simulink model "sampleModel1768_sub"  (R2023a)
settings: Solver=VariableStepAuto  StartTime=0.0  StopTime=10.0  RelTol=1e-3
libraries: hdlsllib x6, simulink x2
settings Model: Creator=user1  LastModifiedBy=user1
settings OptimizationCC: BlockReduction=off  ConditionallyExecuteInputs=off

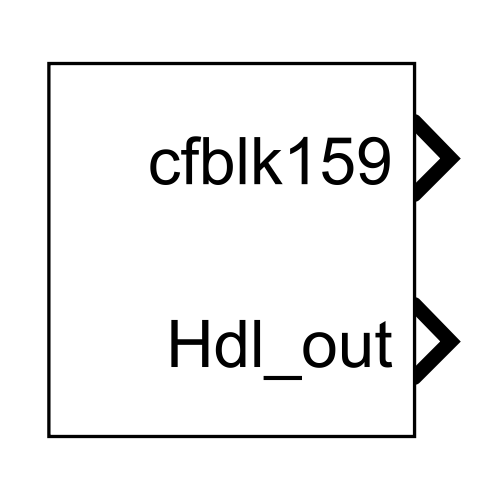
[thumbnail: Simulink's stored preview of the top-level diagram]
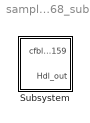
== system sampleModel1768_sub ==
  Subsystem : Subsystem

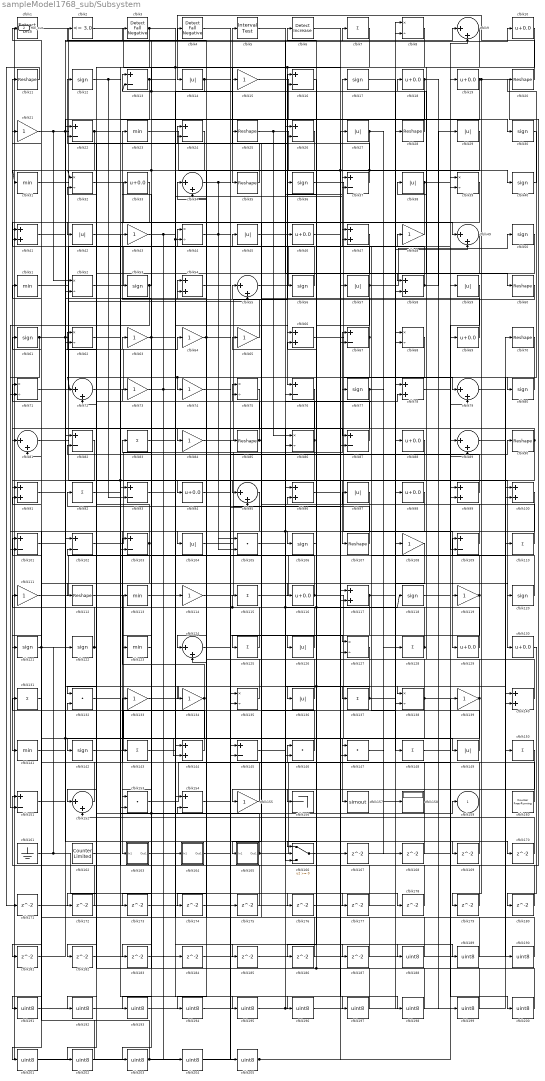
== system sampleModel1768_sub/Subsystem ==
  cfblk1 : simulink/Logic and Bit Operations/Extract Bits  bitsToExtract=Upper half  numBits=8  bitIdxRange=[0 7]  outScalingMode=Preserve fixed-point scaling
      settings: LibrarySourceBlock=|
      | hdlsllib/Logic and Bit
      | Operations/Extract Bits
  cfblk{10,18..19,33,46,69,88,94,98,116,129..130} (12 alike) : Bias  Bias=0.0  SaturateOnIntegerOverflow=off
  cfblk{41,47,54,58,66,78,91,96,99..100,117,140,144} (13 alike) : Sum  OutDataTypeStr=uint8
  cfblk{13,16,22,24,26,37,67,76,82,87,93,101..103,109,145,151,154} (18 alike) : Sum  Inputs=+-  OutDataTypeStr=uint8
  cfblk{14,27,29,38,42,45,57,59,97,104,126,136,149} (13 alike) : Abs  OutDataTypeStr=uint8  SaturateOnIntegerOverflow=off
  cfblk{105,132,146..147,153} (5 alike) : DotProduct  OutDataTypeStr=uint8
  cfblk{12,17,30,36,40,50,53,56,61,77,80,106,118,120..122,142} (17 alike) : Signum
  cfblk{11,20,25,28,35,60,70,85,90,107,112} (11 alike) : Reshape
  cfblk{15,21,43,48,63..65,73..74,84,108,111,114,119,133..134,139,155} (18 alike) : Gain  OutDataTypeStr=uint8
  cfblk{7,83,92,110,115,125,128,131,137,143,148,150} (12 alike) : Sum  Inputs=+  OutDataTypeStr=uint8
  cfblk{23,31,51,113,123,141} (6 alike) : MinMax  OutDataTypeStr=uint8
  cfblk{9,34,49,55,72,79,81,89,95,124,152} (11 alike) : Sum  Inputs=|++  OutDataTypeStr=uint8
  cfblk{8,32,39,44,52,62,68,71,75,86,127,135,138} (13 alike) : Product  Inputs=*/  OutDataTypeStr=uint8  RndMeth=Zero  SaturateOnIntegerOverflow=on
  cfblk156 : Terminator
  cfblk157 : ToWorkspace  VariableName=simout  SaveFormat=Timeseries  SampleTime=-1
  cfblk158 : Display
  cfblk160 : hdlsllib/Sources/Counter Free-Running  NumBits=16  tsamp=-1
  cfblk161 : Ground
  cfblk162 : hdlsllib/Sources/Counter Limited  uplimit=7  tsamp=-1
  cfblk163 : Subsystem
      settings: LibrarySourceBlock=|
      | hdlsllib/Ports &
      | Subsystems/Subsystem
  cfblk164 : Subsystem
      settings: LibrarySourceBlock=|
      | hdlsllib/Ports &
      | Subsystems/Subsystem
  cfblk165 : Subsystem
      settings: LibrarySourceBlock=|
      | hdlsllib/Ports &
      | Subsystems/Subsystem
  cfblk166 : Switch  OutDataTypeStr=uint8  SaturateOnIntegerOverflow=off  InputSameDT=off
  cfblk{167..187} (21 alike) : Delay  SampleTime=1
  cfblk{188..205} (18 alike) : DataTypeConversion  OutDataTypeStr=uint8  SaturateOnIntegerOverflow=off  RndMeth=Floor
  cfblk2 : hdlsllib/Logic and Bit Operations/Compare To Constant  relop=<=  const=3.0  OutDataTypeStr=uint8
  cfblk3 : hdlsllib/Logic and Bit Operations/Detect Fall Negative  vinit=0  OutDataTypeStr=uint8
  cfblk4 : hdlsllib/Logic and Bit Operations/Detect Fall Negative  vinit=0  OutDataTypeStr=uint8
  cfblk5 : hdlsllib/Logic and Bit Operations/Interval Test  IntervalClosedRight=on  uplimit=0.5  IntervalClosedLeft=on  lowlimit=-0.5  OutDataTypeStr=uint8
  cfblk6 : simulink/Logic and Bit Operations/Detect Increase  vinit=0.0  OutDataTypeStr=uint8
      settings: LibrarySourceBlock=|
      | hdlsllib/Logic and Bit
      | Operations/Detect
      | Increase
  cfblk159 : Outport  OutDataTypeStr=uint8  VectorParamsAs1DForOutWhenUnconnected=off
  Hdl_out : Outport  Port=2  OutDataTypeStr=uint8
  wires:
  cfblk71/1 -> cfblk48/1
  cfblk58/1 -> cfblk36/1, cfblk29/1
  cfblk60/1 -> cfblk55/1
  cfblk7/1 -> cfblk123/1, cfblk76/1
  cfblk33/1 -> cfblk141/1
  cfblk20/1 -> cfblk14/1
  cfblk116/1 -> cfblk53/1, cfblk149/1
  cfblk66/1 -> cfblk79/1
  cfblk107/1 -> cfblk92/1
  cfblk30/1 -> cfblk80/1
  cfblk161/1 -> cfblk205/1, cfblk122/1
  cfblk84/1 -> cfblk16/1
  cfblk14/1 -> cfblk187/1, cfblk13/1
  cfblk153/1 -> cfblk146/1
  cfblk104/1 -> cfblk46/1
  cfblk31/1 -> cfblk130/1
  cfblk65/1 -> cfblk23/1
  cfblk64/1 -> cfblk176/1, cfblk4/1
  cfblk1/1 -> cfblk107/1
  cfblk112/1 -> cfblk144/2
  cfblk72/1 -> cfblk64/1
  cfblk24/1 -> cfblk132/1
  cfblk88/1 -> cfblk95/1
  cfblk137/1 -> cfblk49/2, cfblk136/1
  cfblk136/1 -> cfblk111/1
  cfblk121/1 -> cfblk41/1, cfblk63/1
  cfblk100/1 -> cfblk191/1, cfblk166/3
  cfblk57/1 -> cfblk47/2, cfblk126/1, cfblk50/1
  cfblk68/1 -> cfblk193/1
  cfblk147/1 -> cfblk158/1
  cfblk44/1 -> cfblk178/1, cfblk105/1
  cfblk75/1 -> cfblk84/1
  cfblk55/1 -> cfblk19/1
  cfblk19/1 -> cfblk166/1, cfblk179/1, cfblk151/1
  cfblk76/1 -> cfblk104/1
  cfblk165/1(Out1) -> cfblk59/1, cfblk113/1, cfblk132/2
  cfblk2/1 -> cfblk117/1, cfblk154/1
  cfblk139/1 -> cfblk172/1, cfblk56/1
  cfblk108/1 -> cfblk121/1
  cfblk129/1 -> cfblk16/2, cfblk73/1
  cfblk48/1 -> cfblk42/1
  cfblk138/1 -> cfblk200/1, cfblk2/1, cfblk157/1
  cfblk132/1 -> cfblk43/1
  cfblk47/1 -> cfblk106/1
  cfblk61/1 -> cfblk71/2, cfblk86/2, cfblk17/1
  cfblk122/1 -> cfblk192/1, cfblk101/1
  cfblk36/1 -> cfblk129/1
  cfblk133/1 -> cfblk137/1
  cfblk102/1 -> cfblk67/1
  cfblk25/1 -> cfblk86/1, cfblk40/1
  cfblk37/1 -> cfblk31/1, cfblk5/1
  cfblk13/1 -> cfblk62/2, cfblk66/1
  cfblk56/1 -> cfblk11/1
  cfblk39/1 -> cfblk203/1
  cfblk97/1 -> cfblk163/1(In1)
  cfblk86/1 -> cfblk62/1, cfblk153/2, cfblk142/1
  cfblk146/1 -> cfblk75/1
  cfblk109/1 -> cfblk75/2
  cfblk43/1 -> cfblk189/1, cfblk184/1
  cfblk29/1 -> cfblk152/1
  cfblk105/1 -> cfblk37/1
  cfblk51/1 -> cfblk55/2
  cfblk127/1 -> cfblk156/1, cfblk146/2
  cfblk8/1 -> cfblk35/1
  cfblk35/1 -> cfblk12/1
  cfblk28/1 -> cfblk3/1, cfblk13/2
  cfblk151/1 -> cfblk54/1
  cfblk117/1 -> cfblk127/2, cfblk28/1
  cfblk27/1 -> cfblk128/1, cfblk87/2, cfblk173/1, cfblk32/1
  cfblk114/1 -> cfblk27/1
  cfblk41/1 -> cfblk134/1
  cfblk38/1 -> cfblk9/2, cfblk125/1
  cfblk77/1 -> cfblk168/1, cfblk166/2
  cfblk52/1 -> cfblk8/2
  cfblk80/1 -> cfblk72/1, cfblk74/1
  cfblk128/1 -> cfblk38/1, cfblk72/2, cfblk115/1
  cfblk115/1 -> cfblk69/1
  cfblk32/1 -> cfblk78/1
  cfblk70/1 -> cfblk100/2
  cfblk160/1 -> cfblk51/1
  cfblk12/1 -> cfblk93/2, cfblk30/1
  cfblk69/1 -> cfblk44/1
  cfblk81/1 -> cfblk114/1
  cfblk53/1 -> cfblk101/2, cfblk33/1
  cfblk15/1 -> cfblk108/1
  cfblk143/1 -> cfblk37/2
  cfblk21/1 -> cfblk52/1, cfblk9/1, cfblk26/2
  cfblk152/1 -> cfblk21/1
  cfblk144/1 -> cfblk61/1
  cfblk79/1 -> cfblk110/1
  cfblk103/1 -> cfblk182/1, cfblk32/2
  cfblk18/1 -> cfblk199/1, cfblk153/1
  cfblk67/1 -> cfblk194/1, cfblk24/1
  cfblk5/1 -> cfblk60/1
  cfblk140/1 -> cfblk18/1
  cfblk155/1 -> cfblk133/1
  cfblk148/1 -> cfblk139/1
  cfblk94/1 -> cfblk95/2
  cfblk162/1 -> cfblk159/1
  cfblk17/1 -> cfblk119/1
  cfblk150/1 -> cfblk155/1
  cfblk90/1 -> cfblk117/2, cfblk81/1
  cfblk134/1 -> cfblk181/1, cfblk103/1
  cfblk141/1 -> cfblk147/1
  cfblk99/1 -> cfblk82/2
  cfblk120/1 -> cfblk109/1
  cfblk93/1 -> cfblk15/1, cfblk44/2
  cfblk59/1 -> cfblk109/2
  cfblk40/1 -> cfblk20/1
  cfblk119/1 -> cfblk47/1, cfblk165/1(In1)
  cfblk10/1 -> cfblk58/1
  cfblk73/1 -> cfblk204/1, cfblk195/1
  cfblk26/1 -> cfblk124/1
  cfblk3/1 -> cfblk103/2, cfblk164/1(In1)
  cfblk111/1 -> cfblk70/1
  cfblk78/1 -> cfblk79/2
  cfblk164/1(Out1) -> cfblk145/1
  cfblk166/1 -> cfblk98/1
  cfblk23/1 -> cfblk148/1
  cfblk145/1 -> cfblk118/1, cfblk78/2
  cfblk87/1 -> cfblk65/1
  cfblk49/1 -> cfblk94/1
  cfblk125/1 -> cfblk71/1
  cfblk126/1 -> cfblk54/2
  cfblk16/1 -> cfblk116/1
  cfblk142/1 -> cfblk88/1
  cfblk45/1 -> cfblk7/1
  cfblk62/1 -> cfblk87/1
  cfblk82/1 -> cfblk91/1
  cfblk118/1 -> cfblk120/1
  cfblk98/1 -> cfblk151/2
  cfblk63/1 -> cfblk145/2, cfblk143/1
  cfblk96/1 -> cfblk198/1
  cfblk135/1 -> cfblk102/2
  cfblk101/1 -> cfblk170/1, cfblk147/2
  cfblk149/1 -> cfblk97/1
  cfblk154/1 -> cfblk90/1
  cfblk54/1 -> cfblk127/1
  cfblk42/1 -> cfblk140/2
  cfblk110/1 -> cfblk77/1
  cfblk22/1 -> cfblk52/2, cfblk49/1
  cfblk34/1 -> cfblk105/2, cfblk138/1
  cfblk9/1 -> cfblk112/1
  cfblk91/1 -> cfblk10/1
  cfblk85/1 -> cfblk24/2, cfblk25/1
  cfblk124/1 -> cfblk135/1
  cfblk46/1 -> cfblk167/1
  cfblk167/1 -> cfblk99/2
  cfblk168/1 -> cfblk26/1
  cfblk163/1(Out1) -> cfblk169/1
  cfblk169/1 -> cfblk1/1
  cfblk170/1 -> cfblk152/2
  cfblk11/1 -> cfblk171/1
  cfblk171/1 -> cfblk138/2
  cfblk172/1 -> cfblk81/2
  cfblk173/1 -> cfblk135/2
  cfblk95/1 -> cfblk174/1
  cfblk174/1 -> cfblk154/2
  cfblk74/1 -> cfblk175/1
  cfblk175/1 -> cfblk124/2
  cfblk176/1 -> cfblk8/1
  cfblk4/1 -> cfblk177/1
  cfblk177/1 -> cfblk22/1
  cfblk178/1 -> cfblk34/1
  cfblk179/1 -> cfblk93/1
  cfblk130/1 -> cfblk180/1
  cfblk180/1 -> cfblk102/1
  cfblk181/1 -> cfblk82/1
  cfblk182/1 -> cfblk140/1
  cfblk123/1 -> cfblk183/1
  cfblk183/1 -> cfblk100/1
  cfblk184/1 -> cfblk58/2
  cfblk113/1 -> cfblk185/1
  cfblk185/1 -> cfblk67/2
  cfblk106/1 -> cfblk186/1
  cfblk186/1 -> cfblk144/1
  cfblk187/1 -> cfblk91/2
  cfblk6/1 -> cfblk188/1
  cfblk188/1 -> cfblk45/1
  cfblk189/1 -> cfblk6/1
  cfblk89/1 -> cfblk190/1
  cfblk190/1 -> cfblk34/2
  cfblk191/1 -> cfblk89/1
  cfblk192/1 -> cfblk89/2
  cfblk193/1 -> cfblk76/2, cfblk150/1
  cfblk194/1 -> cfblk68/1
  cfblk195/1 -> cfblk68/2
  cfblk83/1 -> cfblk196/1
  cfblk196/1 -> cfblk99/1
  cfblk92/1 -> cfblk197/1
  cfblk197/1 -> cfblk83/1
  cfblk198/1 -> cfblk66/2, cfblk22/2
  cfblk199/1 -> cfblk96/1
  cfblk200/1 -> cfblk96/2
  cfblk131/1 -> cfblk201/1
  cfblk201/1 -> cfblk85/1
  cfblk50/1 -> cfblk202/1
  cfblk202/1 -> cfblk131/1
  cfblk203/1 -> cfblk57/1, cfblk41/2
  cfblk204/1 -> cfblk39/1
  cfblk205/1 -> Hdl_out/1, cfblk39/2

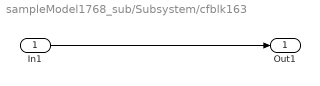
== system sampleModel1768_sub/Subsystem/cfblk163 ==
  In1 : Inport
  Out1 : Outport
  wires:
  In1/1 -> Out1/1

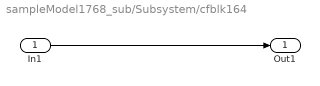
== system sampleModel1768_sub/Subsystem/cfblk164 ==
  In1 : Inport
  Out1 : Outport
  wires:
  In1/1 -> Out1/1

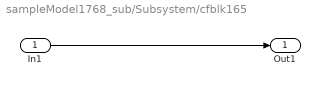
== system sampleModel1768_sub/Subsystem/cfblk165 ==
  In1 : Inport
  Out1 : Outport
  wires:
  In1/1 -> Out1/1
